simulink model "EEE4022S_Single_Pendulum_lsqnonlin"  (R2021a)
settings: Solver=ode4  StartTime=0.0  StopTime=100  FixedStep=0.002  RelTol=1e-3
undefined symbols (not defined in the file or in its folder): B_p, J_p
libraries: simulink_extras x1
settings Model: Creator=User  LastModifiedBy=User
settings SolverCC: AutoInsertRateTranBlk=on

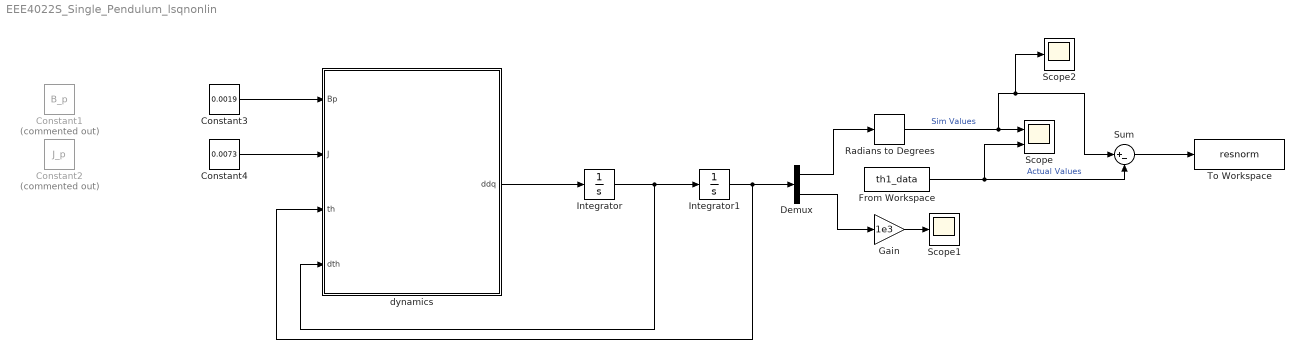
== system EEE4022S_Single_Pendulum_lsqnonlin ==
  Constant1 : Constant  Commented=on  Value=B_p
  Constant2 : Constant  Commented=on  Value=J_p
  Constant3 : Constant  Value=0.0019
  Constant4 : Constant  Value=0.0073
  Demux : Demux  Outputs=2
  From Workspace : FromWorkspace  VariableName=th1_data  SampleTime=0.002
  Gain : Gain  Gain=1e3
  Integrator : Integrator  InitialCondition=[0 0]
  Integrator1 : Integrator  InitialCondition=[10*pi/180 0]
  Radians to Degrees : simulink_extras/Transformations/Radians to Degrees
  Scope : Scope  NumInputPorts=2
  Scope1 : Scope
  Scope2 : Scope
  Sum : Sum  Inputs=|+-
  To Workspace : ToWorkspace  VariableName=resnorm  SaveFormat=Timeseries  SampleTime=0.002
  dynamics : MATLAB Function  TreatAsAtomicUnit=on
  wires:
  Integrator/1 -> dynamics/4(dth), Integrator1/1
  dynamics/1(ddq) -> Integrator/1
  Integrator1/1 -> dynamics/3(th), Demux/1
  Demux/1 -> Radians to Degrees/1
  Demux/2 -> Gain/1
  Radians to Degrees/1 -> Scope2/1, Sum/1, Scope/1  "Sim Values"
  Gain/1 -> Scope1/1
  Constant3/1 -> dynamics/1(Bp)
  Constant4/1 -> dynamics/2(J)
  From Workspace/1 -> Sum/2, Scope/2  "Actual Values"
  Sum/1 -> To Workspace/1

== matlab function EEE4022S_Single_Pendulum_lsqnonlin/dynamics ==
  data: Bp input; J input; th input; dth input; ddq output
function ddq = dynamics(Bp,J,th,dth)
%#codegen

%    This function was generated by the Symbolic Math Toolbox version 8.7.
%    25-Oct-2022 13:27:13

g = 9.81;
m = 0.230;
l = 0.3302;

sgn = 0;
Cp = 0;

ddq = -(Bp.*dth+Cp.*sgn+g.*l.*m.*sin(th))./(J+l.^2.*m);
